simulink model "Geneva_Drive"  (R2017a)
settings: Solver=ode15s  StartTime=0.0  StopTime=30  MaxStep=1e-2  RelTol=1e-4  AbsTol=1e-5  EnableMultiTasking=on
PostLoadFcn:
  | set_param(bdroot,'IgnoredZcDiagnostic','none')
  | warning off sm:compiler:topologyAnalysis:DanglingBlock
StartFcn:
  | tic;
StopFcn:
  | Elapsed_Sim_Time = toc;
  | disp(['Elapsed Sim Time = ' num2str(Elapsed_Sim_Time)]);
undefined symbols (not defined in the file or in its folder): X, Y, Z
libraries: sm_lib x44, Contact_Forces_Lib x20, nesl_utility x5, simulink x1
(part 1 of 2)
CloseFcn:
  | try,close(h1_Geneva_Drive),end
  | clear h1_Geneva_Drive
  | 
  | clear simlog_Geneva_Drive
Description:
  | Geneva Drive
  | 
  | Copyright 2015-2017 The MathWorks, Inc.
settings Model: Creator=smiller  LastModifiedBy=smiller
settings DataIOCC: MaxDataPoints=15000  SaveFormat=StructureWithTime  SaveState=on  SignalLoggingName=logsout_Geneva_Drive
settings OptimizationCC: LifeSpan=inf
settings DebuggingCC: IgnoredZcDiagnostic=none  SolverPrmCheckMsg=warning  AllowSymbolicDim=off  SFUnexpectedBacktrackingDiag=warning  SFNoUnconditionalDefaultTransitionDiag=warning  SFExecutionAtInitializationDiag=none
settings HardwareCC: ProdBitPerPointer=32  ProdBitPerSizeT=32  ProdBitPerPtrDiffT=32  ProdLargestAtomicFloat=None  ProdIntDivRoundTo=Undefined  ProdEndianess=Unspecified  ProdWordSize=32  ProdHWDeviceType=32-bit Generic
settings ModelReferenceCC: PropagateSignalLabelsOutOfModel=off
settings GRTTargetCC: TargetLangStandard=C89/C90 (ANSI)  GeneratePreprocessorConditionals=Disable all
settings ConfigComp: CovMetricSettings=dw  CovHtmlReporting=on  CovSaveCumulativeToWorkspaceVar=on  CovSaveSingleToWorkspaceVar=on  CovExternalEMLEnable=off  CovSFcnEnable=off
settings SimscapeCC: SimscapeLogType=all  SimscapeLogSimulationStatistics=on  SimscapeLogName=simlog_Geneva_Drive  SimscapeLogDataHistory=15000
settings ConfigurationSet: Description=SimMechanics 2G
settings ExplorerConfigSet: InternalSimMechanicsExplorerSettings="<ExplorerConfiguration><canonicalview>default</canonicalview><AnimationSetting><BasePlaybackSpeed>1.0</BasePlaybackSpeed><PlaybackSpeedFactor>4.0</PlaybackSpeedFactor></AnimationSetting><TilePanel><TileInfo><Tiles Columns=\"1\" Count=\"1\" Rows=\"1\"><Column Left=\"2\" Weight=\"1\"/><Column Left=\"677\"/><Row Top=\"2\" Weight=\"1\"/><Row Top=\"558\"/><Tile Height=\"1\" Width=\"1\" X=\"0\" Y=\"0\"/></Tiles></TileInfo><SceneInfo><SceneViewer><BGColor><R>0.93725490570068359</R><G>0.9686274528503418</G><B>0.9686274528503418</B></BGColor><Camera><Position><X>0.26080521668652706</X><Y>0.4639017710068058</Y><Z>0.36701914488687676</Z></Position><Center><X>-0.034093618327655228</X><Y>0.025639318022065816</Y><Z>-0.010275526182887462</Z></Center><Up><X>-0.45579088703273962</X><Y>0.73671340761661774</Y><Z>-0.4995077800553458</Z></Up><Left>-0.33774445205926895</Left><Right>0.33774445205926895</Right><Bottom>-0.208832748234272</Bottom><Top>0.208832748234272</Top></Camera></SceneViewer></SceneInfo></TilePanel></ExplorerConfiguration>"

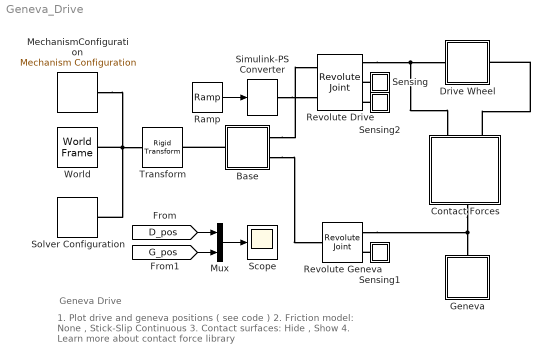
== system Geneva_Drive ==
  note: 1. Plot drive and geneva positions ( see code )
      | 2. Friction model: None , Stick-Slip Continuous
      | 3. Contact surfaces: Hide , Show
      | 4. Learn more about contact force library
  note: Geneva Drive
  Base : Subsystem
  Contact Forces : Subsystem
  Drive Wheel : Subsystem  Tag=CustomStyle
  Geneva : Subsystem  Tag=CustomStyle
  MechanismConfiguration : sm_lib/Utilities/Mechanism Configuration  UniformGravity=Constant  GravityVector=[0 -9.81 0]  GravityUnits=m/s^2  LinearizationDelta=0.001
  Mux : Mux  Inputs=2
  Ramp : simulink/Sources/Ramp  slope=72  start=0  X0=106.26478005487978
  Revolute Drive : sm_lib/Joints/Revolute Joint  SenseConstraintForce=off  SenseConstraintForceX=off  SenseConstraintForceY=off  SenseConstraintForceZ=off  SenseConstraintTorque=off  SenseConstraintTorqueX=off  SenseConstraintTorqueY=off  SenseConstraintTorqueZ=off  SenseTotalForce=off  SenseTotalForceX=off  SenseTotalForceY=off  SenseTotalForceZ=off  SenseTotalTorque=off  SenseTotalTorqueX=off  SenseTotalTorqueY=off  SenseTotalTorqueZ=off  CompositeWrenchDir=FollowerOnBase  CompositeWrenchFrame=BaseFrame  EquilibriumPosition=0  EquilibriumPositionUnits=rad  SpringStiffness=0  SpringStiffnessUnits=m*N/rad  DampingCoefficient=0  DampingCoefficientUnits=m*s*N/rad  TorqueActuationMode=ComputedTorque  MotionActuationMode=InputMotion  SensePosition=on  SenseVelocity=off  SenseAcceleration=off  SenseTorqueForce=on  PositionTargetSpecify=on  PositionTargetPriority=Low  PositionTargetValue=106.26478005487978  PositionTargetValueUnits=deg  VelocityTargetSpecify=off  VelocityTargetPriority=High  VelocityTargetValue=0  VelocityTargetValueUnits=deg/s
  Revolute Geneva : sm_lib/Joints/Revolute Joint  SenseConstraintForce=off  SenseConstraintForceX=off  SenseConstraintForceY=off  SenseConstraintForceZ=off  SenseConstraintTorque=off  SenseConstraintTorqueX=off  SenseConstraintTorqueY=off  SenseConstraintTorqueZ=off  SenseTotalForce=off  SenseTotalForceX=off  SenseTotalForceY=off  SenseTotalForceZ=off  SenseTotalTorque=off  SenseTotalTorqueX=off  SenseTotalTorqueY=off  SenseTotalTorqueZ=off  CompositeWrenchDir=FollowerOnBase  CompositeWrenchFrame=BaseFrame  EquilibriumPosition=90.000000000003197  EquilibriumPositionUnits=deg  SpringStiffness=0  SpringStiffnessUnits=m*N/rad  DampingCoefficient=1  DampingCoefficientUnits=m*s*N/rad  TorqueActuationMode=NoTorque  MotionActuationMode=ComputedMotion  SensePosition=on  SenseVelocity=off  SenseAcceleration=off  SenseTorqueForce=off  PositionTargetSpecify=on  PositionTargetPriority=Low  PositionTargetValue=90.000000000003197  PositionTargetValueUnits=deg  VelocityTargetSpecify=off  VelocityTargetPriority=High  VelocityTargetValue=0  VelocityTargetValueUnits=deg/s
  Scope : Scope
  Sensing : Subsystem  Tag=CustomStyle
  Sensing1 : Subsystem  Tag=CustomStyle
  Sensing2 : Subsystem
  Simulink-PS Converter : nesl_utility/Simulink-PS Converter  PhysicalDomain=network_engine_domain  SubClassName=ps_input  LeftPortType=input  RightPortType=output  PseudoPeriodic=off  Frequencies=[]  NoiseDistribution=none  NoiseParameters=[]  Unit=deg  AffineConversion=off  FilteringAndDerivatives=filter  SimscapeFilterOrder=2  InputFilterTimeConstant=0.01  UdotUserProvided=1
  Solver Configuration : nesl_utility/Solver Configuration  PhysicalDomain=network_engine_domain  SubClassName=solver  LeftPortType=input  RightPortType=generic  Accelerate=off  Tones=[]  Harmonics=[]  SimulateNoise=off  Profile=off  UseLocalSampling=off  EnableSwitchedLinearOptims=on  FrequencyDomain=off  UseCCode=off  RelTol=0.001  AbsTol=1e-06  MinStep=1e-09  ToWorkspace=off  RevertToSquareIcSolve=off  NumHomotopyIterations=100  PhasorMode=off  PhasorModeNumHarmonics=1  OverrideAbsTol=off  DoDC=off  ResidualTolerance=1e-09  UseLocalSolver=off  LocalSolverChoice=NE_BACKWARD_EULER_ADVANCER  LocalSolverSampleTime=0.001  DoFixedCost=off  MaxNonlinIter=3  MaxModeIter=2  LinearAlgebra=Sparse  DelaysMemoryBudget=1024  AutomaticFiltering=on  FilteringTimeConstant=0.001
  "Transform " : sm_lib/Frames and Transforms/Rigid Transform  TranslationMethod=Cartesian  TranslationStandardOffset=0  TranslationLengthUnit=mm  TranslationStandardAxis=+Z  TranslationCartesianOffset=[-30.994181557875464 40 -14.83110487348719]  TranslationROffset=0  TranslationROffsetUnits=m  TranslationZOffset=0  TranslationZOffsetUnits=m  TranslationThetaOffset=0  TranslationThetaOffsetUnits=deg  RotationMethod=ArbitraryAxis  RotationAngleUnits=rad  RotationStandardAxis=+Z  RotationAngle=1.5707963267948966  RotationArbitraryAxis=[-1 0 0]  FollAlignAxisA=+X  BaseAlignAxisA=+Y  FollAlignAxisB=+Y  BaseAlignAxisB=+Z  RotationSequenceAxes=FollowerAxes  RotationSequence=XYX  RotationSequenceAngles=[0 0 0]  RotationSequenceAnglesUnits=deg  RotationMatrix=[1 0 0; 0 1 0; 0 0 1]
  World : sm_lib/Frames and Transforms/World Frame
  wires:
  Ramp/1 -> Simulink-PS Converter/1
  [D_pos] -> Mux/1
  Mux/1 -> Scope/1
  [G_pos] -> Mux/2
  connections:
  World/RConn1 -- MechanismConfiguration/RConn1 -- "Transform "/LConn1 -- Solver Configuration/RConn1
  Revolute Drive/RConn1 -- Drive Wheel/LConn1 -- Contact Forces/RConn1
  Revolute Geneva/RConn1 -- Geneva/LConn1 -- Contact Forces/LConn1
  Sensing2/LConn1 -- Revolute Drive/RConn3
  Sensing1/LConn1 -- Revolute Geneva/RConn2
  Sensing/LConn1 -- Revolute Drive/RConn2
  Contact Forces/RConn2 -- Drive Wheel/RConn1
  Simulink-PS Converter/RConn1 -- Revolute Drive/LConn2
  Base/LConn1 -- "Transform "/RConn1
  Base/RConn1 -- Revolute Drive/LConn1
  Base/RConn2 -- Revolute Geneva/LConn1

== system Geneva_Drive/Base ==
  ReferenceFrame : sm_lib/Frames and Transforms/Reference Frame
  Solid : sm_lib/Body Elements/Solid  InertiaType=Custom  Mass=5.6121441650895836  MassUnits=kg  CenterOfMass=[0.22415415704528135 0 -24.782168314450626]  CenterOfMassUnits=mm  MomentsOfInertia=[57246.923822174664 131168.16755878026 187513.90774897448]  MomentsOfInertiaUnits=kg*mm^2  ProductsOfInertia=[0 -24.879239071091789 0]  ProductsOfInertiaUnits=kg*mm^2  DensityBased=on  Density=1000  DensityUnits=kg/(m^3)  DoExposeReferenceFrame=on  SerializedFrames=<Frames/>  GraphicType=FromGeometry  MarkerShape=Sphere  MarkerSize=10  MarkerSizeUnits=m  GraphicVisPropType=SimpleVisualProperties  GraphicDiffuseColor=[0.82745098039215681 0.82745098039215681 0.81960784313725488]  GraphicSpecularColor=[0.5 0.5 0.5 1.0]  GraphicAmbientColor=[0.15 0.15 0.15 1.0]  GraphicEmissiveColor=[0.0 0.0 0.0 1.0]  GraphicShininess=75  GraphicOpacity=1  GeometryShape=FromFile  RectangleSize=[1 1]  RectangleSizeUnits=m  BrickDimensions=[1 1 1]  BrickDimensionUnits=m  CylinderRadius=1  CylinderRadiusUnits=m  CylinderLength=1  CylinderLengthUnits=m  SphereRadius=1  SphereRadiusUnits=m  EllipsoidRadii=[1 1 1]  EllipsoidRadiiUnits=m  ExtrusionCrossSection=[1 1; -1 1; -1 -1; 1 -1]  ExtrusionCrossSectionUnits=m  ExtrusionLength=1  ExtrusionLengthUnits=m  PolygonNumSides=3  PolygonOuterRadius=1  PolygonOuterRadiusUnits=m  ExtGeomFileType=STL  ExtGeomFileName=Base_Default_sldprt.STL  ExtGeomFileUnits=mm  RevolutionCrossSection=[1 1; 1 -1; 2 -1; 2 1]  RevolutionCrossSectionUnits=m  RevolutionExtent=Full  RevolutionAngle=180  RevolutionAngleUnits=deg
  Transform : sm_lib/Frames and Transforms/Rigid Transform  TranslationMethod=Cartesian  TranslationStandardOffset=0  TranslationLengthUnit=mm  TranslationStandardAxis=+Z  TranslationCartesianOffset=[100 0 0]  TranslationROffset=0  TranslationROffsetUnits=m  TranslationZOffset=0  TranslationZOffsetUnits=m  TranslationThetaOffset=0  TranslationThetaOffsetUnits=deg  RotationMethod=ArbitraryAxis  RotationAngleUnits=rad  RotationStandardAxis=+Z  RotationAngle=0  RotationArbitraryAxis=[0 0 0]  FollAlignAxisA=+X  BaseAlignAxisA=+Y  FollAlignAxisB=+Y  BaseAlignAxisB=+Z  RotationSequenceAxes=FollowerAxes  RotationSequence=XYX  RotationSequenceAngles=[0 0 0]  RotationSequenceAnglesUnits=deg  RotationMatrix=[1 0 0; 0 1 0; 0 0 1]
  Transform2 : sm_lib/Frames and Transforms/Rigid Transform  TranslationMethod=Cartesian  TranslationStandardOffset=0  TranslationLengthUnit=mm  TranslationStandardAxis=+Z  TranslationCartesianOffset=[-99.999999999999986 0 57.42640687119286*0]  TranslationROffset=0  TranslationROffsetUnits=m  TranslationZOffset=0  TranslationZOffsetUnits=m  TranslationThetaOffset=0  TranslationThetaOffsetUnits=deg  RotationMethod=ArbitraryAxis  RotationAngleUnits=rad  RotationStandardAxis=+Z  RotationAngle=3.1415926535897931  RotationArbitraryAxis=[1 0 0]  FollAlignAxisA=+X  BaseAlignAxisA=+Y  FollAlignAxisB=+Y  BaseAlignAxisB=+Z  RotationSequenceAxes=FollowerAxes  RotationSequence=XYX  RotationSequenceAngles=[0 0 0]  RotationSequenceAnglesUnits=deg  RotationMatrix=[1 0 0; 0 1 0; 0 0 1]
  F3 : PMIOPort  Port=1  Side=Left
  F2 : PMIOPort  Port=2  Side=Right
  F : PMIOPort  Port=3  Side=Right
  connections:
  Transform2/RConn1 -- F2/RConn1
  Transform/RConn1 -- F/RConn1
  F3/RConn1 -- Transform2/LConn1 -- Transform/LConn1 -- ReferenceFrame/RConn1 -- Solid/RConn1

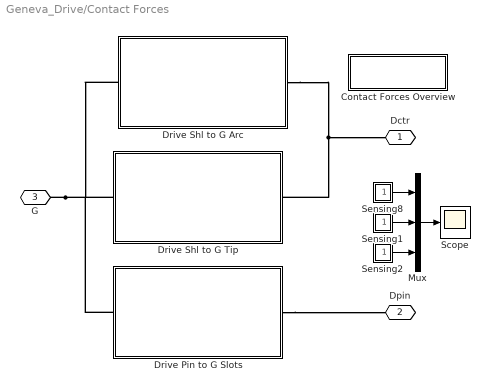
== system Geneva_Drive/Contact Forces ==
  Contact Forces Overview : Subsystem
      settings: OpenFcn=web(which('Geneva_Drive_Contact_Forces.html'));
      mask Display: disp('Contact Forces\nOverview');
  Drive Pin to G Slots : Subsystem  mask(Contact Forces, Drive Pin and Geneva Slot){r_drive_pin=0.015, l_genv_lin=0.1405*2, k_contact=1e5, b_contact=1e4, d_genv_lin=0.0055, vis_len_genevadrive=0.03, vis_dep_genevadrive=0.001}
      mask prompts: r_drive_pin "Radius of Drive Wheel Pin (m)"; l_genv_lin "Slot Length Through Geneva (m)"; k_contact "Contact Stiffness (N/m)"; b_contact "Contact Damping (N/(m/s))"; d_genv_lin "Line Thickness, Geneva Slot (m)"; vis_len_genevadrive "Contact Surface Visualization Height(m)"; vis_dep_genevadrive "Contact Surface Visualization Thickness (m)"
      mask help:
      | This subsystem models the contact forces between the drive wheel pin and the four slots on the Geneva.  All contact forces are identical.  They connect one reference frame on the drive wheel pin and four reference frames on the Geneva.
      |
      | Click the Help button for a diagram of the contact forces and the parameters.
      mask Help: web(which('Geneva_Drive_Contact_DPin_GSlot.html'));
      mask Display:
      | image(imread('Contact_Diagram_Dpin_to_GSlot_IMAGE.jpg'));
      | port_label('LConn',1,'LinB');
      | port_label('RConn',1,'CirF');
  Drive Shl to G Arc : Subsystem  mask(Contact Forces, Drive Shoulder and Geneva Arc){r_shld_cir=0.005, r_genv_xcir=0.115, d_genv_ctr_to_xcir=0.2, k_contact=1e4, b_contact=1e2, d_genv_xcir=0.005, vis_len_genevadrive=0.03, vis_dep_genevadrive=0.001}
      mask prompts: r_shld_cir "Circle Radius, Drive Wheel Shoulder (m)"; r_genv_xcir "Ring Radius, Geneva Arc (m)"; d_genv_ctr_to_xcir "Distance Geneva axis to center exterior circle (m)"; k_contact "Contact Stiffness (N/m)"; b_contact "Contact Damping (N/(m/s))"; d_genv_xcir "Ring Thickness, Geneva Arc (m)"; vis_len_genevadrive "Contact Surface Visualization Height(m)"; vis_dep_genevadrive "Contact Surface Visualization Thickness (m)"
      mask help:
      | This subsystem models the contact forces between the drive wheel shoulder and the exterior arcs on the Geneva.  All contact forces are identical.  They connect two reference frames on the drive wheel and four reference frames on the Geneva.
      |
      | Click the Help button for a diagram of the contact forces and the parameters.
      mask Help: web(which('Geneva_Drive_Contact_Shld_Garc.html'));
      mask Display:
      | image(imread('Contact_Diagram_Shld_to_GArc_IMAGE.jpg'));
      | port_label('Lconn',1,'RinB');
      | port_label('Rconn',1,'CirF');
  Drive Shl to G Tip : Subsystem  mask(Contact Forces, Drive Shoulder and Geneva Tips){r_genv_cir=0.0045, r_shld=0.115, k_contact=1e4, b_contact=1e2, d_shld=0.005, vis_len_genevadrive=0.03, vis_dep_genevadrive=0.001}
      mask prompts: r_genv_cir "Circle Radius, Geneva Tip Contact (m)"; r_shld "Ring Radius, Drive Wheel Shoulder (m)"; k_contact "Contact Stiffness (N/m)"; b_contact "Contact Damping (N/(m/s))"; d_shld "Ring Thickness, Drive Wheel Shoulder (m)"; vis_len_genevadrive "Contact Surface Visualization Height(m)"; vis_dep_genevadrive "Contact Surface Visualization Thickness (m)"
      mask help:
      | This subsystem models the contact forces between the drive wheel shoulder and the tips of the Geneva.  All contact forces are identical.  They connect one reference frame on the drive wheel and eight reference frames on the Geneva.
      |
      | Click the Help button for a diagram of the contact forces and the parameters.
      mask Help: web(which('Geneva_Drive_Contact_Shld_Gtip.html'));
      mask Display:
      | image(imread('Contact_Diagram_Gtip_to_Shld_IMAGE.jpg'));
      | port_label('Lconn',1,'CirF');
      | port_label('Rconn',1,'RinB');
  Mux : Mux  Inputs=3
  Scope : Scope
  Sensing1 : Subsystem
  Sensing2 : Subsystem
  Sensing8 : Subsystem
  Dctr : PMIOPort  Port=1  Side=Right
  Dpin : PMIOPort  Port=2  Side=Right
  G : PMIOPort  Port=3  Side=Left
  wires:
  Mux/1 -> Scope/1
  Sensing2/1(S) -> Mux/3
  Sensing1/1(S) -> Mux/2
  Sensing8/1(S) -> Mux/1
  connections:
  G/RConn1 -- Drive Shl to G Arc/LConn1 -- Drive Pin to G Slots/LConn1 -- Drive Shl to G Tip/LConn1
  Drive Pin to G Slots/RConn1 -- Dpin/RConn1
  Drive Shl to G Arc/RConn1 -- Dctr/RConn1 -- Drive Shl to G Tip/RConn1

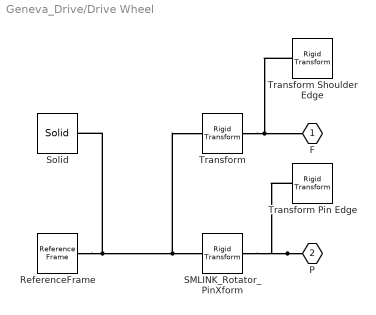
== system Geneva_Drive/Drive Wheel ==
  ReferenceFrame : sm_lib/Frames and Transforms/Reference Frame
  SMLINK_Rotator_PinXform : sm_lib/Frames and Transforms/Rigid Transform  TranslationMethod=Cartesian  TranslationStandardOffset=0  TranslationLengthUnit=mm  TranslationStandardAxis=+Z  TranslationCartesianOffset=[0 99.999999999999943 1.0000000000000009]  TranslationROffset=0  TranslationROffsetUnits=m  TranslationZOffset=0  TranslationZOffsetUnits=m  TranslationThetaOffset=0  TranslationThetaOffsetUnits=deg  RotationMethod=StandardAxis  RotationAngleUnits=deg  RotationStandardAxis=+Z  RotationAngle=10  RotationArbitraryAxis=[0 0 1]  FollAlignAxisA=+X  BaseAlignAxisA=+Y  FollAlignAxisB=+Y  BaseAlignAxisB=+Z  RotationSequenceAxes=FollowerAxes  RotationSequence=XYX  RotationSequenceAngles=[0 0 0]  RotationSequenceAnglesUnits=deg  RotationMatrix=[1 0 0; 0 1 0; 0 0 1]
  Solid : sm_lib/Body Elements/Solid  InertiaType=Custom  Mass=1.1459440199505517  MassUnits=kg  CenterOfMass=[-103.32572655678197 -3.3257265567819814 0.56035000006051983]  CenterOfMassUnits=mm  MomentsOfInertia=[5063.1142307875289 5063.1142307875298 10008.151794093599]  MomentsOfInertiaUnits=kg*mm^2  ProductsOfInertia=[46.956086417341879 46.956086417341901 41.94861289102812]  ProductsOfInertiaUnits=kg*mm^2  DensityBased=on  Density=1000  DensityUnits=kg/(m^3)  DoExposeReferenceFrame=on  SerializedFrames=<Frames/>  GraphicType=FromGeometry  MarkerShape=Sphere  MarkerSize=10  MarkerSizeUnits=m  GraphicVisPropType=SimpleVisualProperties  GraphicDiffuseColor=[0.2 0.4 1.0]  GraphicSpecularColor=[0.5 0.5 0.5 1.0]  GraphicAmbientColor=[0.15 0.15 0.15 1.0]  GraphicEmissiveColor=[0.0 0.0 0.0 1.0]  GraphicShininess=75  GraphicOpacity=1  GeometryShape=FromFile  RectangleSize=[1 1]  RectangleSizeUnits=m  BrickDimensions=[1 1 1]  BrickDimensionUnits=m  CylinderRadius=1  CylinderRadiusUnits=m  CylinderLength=1  CylinderLengthUnits=m  SphereRadius=1  SphereRadiusUnits=m  EllipsoidRadii=[1 1 1]  EllipsoidRadiiUnits=m  ExtrusionCrossSection=[1 1; -1 1; -1 -1; 1 -1]  ExtrusionCrossSectionUnits=m  ExtrusionLength=1  ExtrusionLengthUnits=m  PolygonNumSides=3  PolygonOuterRadius=1  PolygonOuterRadiusUnits=m  ExtGeomFileType=STL  ExtGeomFileName=Drive_Wheel_Default_sldprt.STL  ExtGeomFileUnits=mm  RevolutionCrossSection=[1 1; 1 -1; 2 -1; 2 1]  RevolutionCrossSectionUnits=m  RevolutionExtent=Full  RevolutionAngle=180  RevolutionAngleUnits=deg
  Transform : sm_lib/Frames and Transforms/Rigid Transform  TranslationMethod=Cartesian  TranslationStandardOffset=0  TranslationLengthUnit=mm  TranslationStandardAxis=+Z  TranslationCartesianOffset=[-100.00000000000026 2.1316282072803006e-14 57.426406871192782*0]  TranslationROffset=0  TranslationROffsetUnits=m  TranslationZOffset=0  TranslationZOffsetUnits=m  TranslationThetaOffset=0  TranslationThetaOffsetUnits=deg  RotationMethod=ArbitraryAxis  RotationAngleUnits=rad  RotationStandardAxis=+Z  RotationAngle=3.1415926535897931  RotationArbitraryAxis=[-1 5.9163189700902024e-33 -6.6609835156154749e-17]  FollAlignAxisA=+X  BaseAlignAxisA=+Y  FollAlignAxisB=+Y  BaseAlignAxisB=+Z  RotationSequenceAxes=FollowerAxes  RotationSequence=XYX  RotationSequenceAngles=[0 0 0]  RotationSequenceAnglesUnits=deg  RotationMatrix=[1 0 0; 0 1 0; 0 0 1]
  Transform Pin Edge : sm_lib/Frames and Transforms/Rigid Transform  TranslationMethod=StandardAxis  TranslationStandardOffset=0.015  TranslationLengthUnit=m  TranslationStandardAxis=+X  TranslationCartesianOffset=[0 0 0]  TranslationROffset=0.115  TranslationROffsetUnits=m  TranslationZOffset=0  TranslationZOffsetUnits=m  TranslationThetaOffset=270  TranslationThetaOffsetUnits=deg  RotationMethod=None  RotationAngleUnits=deg  RotationStandardAxis=+Z  RotationAngle=0  RotationArbitraryAxis=[0 0 1]  FollAlignAxisA=+X  BaseAlignAxisA=+Y  FollAlignAxisB=+Y  BaseAlignAxisB=+Z  RotationSequenceAxes=FollowerAxes  RotationSequence=XYX  RotationSequenceAngles=[0 0 0]  RotationSequenceAnglesUnits=deg  RotationMatrix=[1 0 0; 0 1 0; 0 0 1]
  Transform Shoulder Edge : sm_lib/Frames and Transforms/Rigid Transform  TranslationMethod=Cylindrical  TranslationStandardOffset=0.115  TranslationLengthUnit=m  TranslationStandardAxis=+X  TranslationCartesianOffset=[0 0 0]  TranslationROffset=0.115  TranslationROffsetUnits=m  TranslationZOffset=0  TranslationZOffsetUnits=m  TranslationThetaOffset=270  TranslationThetaOffsetUnits=deg  RotationMethod=None  RotationAngleUnits=deg  RotationStandardAxis=+Z  RotationAngle=0  RotationArbitraryAxis=[0 0 1]  FollAlignAxisA=+X  BaseAlignAxisA=+Y  FollAlignAxisB=+Y  BaseAlignAxisB=+Z  RotationSequenceAxes=FollowerAxes  RotationSequence=XYX  RotationSequenceAngles=[0 0 0]  RotationSequenceAnglesUnits=deg  RotationMatrix=[1 0 0; 0 1 0; 0 0 1]
  F : PMIOPort  Port=1  Side=Left
  P : PMIOPort  Port=2  Side=Right
  connections:
  Transform Shoulder Edge/LConn1 -- F/RConn1 -- Transform/RConn1
  P/RConn1 -- Transform Pin Edge/LConn1 -- SMLINK_Rotator_PinXform/RConn1
  ReferenceFrame/RConn1 -- Solid/RConn1 -- Transform/LConn1 -- SMLINK_Rotator_PinXform/LConn1

== system Geneva_Drive/Geneva ==
  ReferenceFrame : sm_lib/Frames and Transforms/Reference Frame
  Solid : sm_lib/Body Elements/Solid  InertiaType=Custom  Mass=0.24105441419713447  MassUnits=kg  CenterOfMass=[100.00000000000023 1.1564451014440063e-12 5.0000000000000009]  CenterOfMassUnits=mm  MomentsOfInertia=[803.62795532691052 803.62795532691234 1603.261580672231]  MomentsOfInertiaUnits=kg*mm^2  ProductsOfInertia=[0 0 0]  ProductsOfInertiaUnits=kg*mm^2  DensityBased=on  Density=1000  DensityUnits=kg/(m^3)  DoExposeReferenceFrame=on  SerializedFrames=<Frames/>  GraphicType=FromGeometry  MarkerShape=Sphere  MarkerSize=10  MarkerSizeUnits=m  GraphicVisPropType=SimpleVisualProperties  GraphicDiffuseColor=[1.0 0.4 0.0]  GraphicSpecularColor=[0.5 0.5 0.5 1.0]  GraphicAmbientColor=[0.15 0.15 0.15 1.0]  GraphicEmissiveColor=[0.0 0.0 0.0 1.0]  GraphicShininess=75  GraphicOpacity=1  GeometryShape=FromFile  RectangleSize=[1 1]  RectangleSizeUnits=m  BrickDimensions=[1 1 1]  BrickDimensionUnits=m  CylinderRadius=1  CylinderRadiusUnits=m  CylinderLength=1  CylinderLengthUnits=m  SphereRadius=1  SphereRadiusUnits=m  EllipsoidRadii=[1 1 1]  EllipsoidRadiiUnits=m  ExtrusionCrossSection=[1 1; -1 1; -1 -1; 1 -1]  ExtrusionCrossSectionUnits=m  ExtrusionLength=1  ExtrusionLengthUnits=m  PolygonNumSides=3  PolygonOuterRadius=1  PolygonOuterRadiusUnits=m  ExtGeomFileType=STL  ExtGeomFileName=Geneva_Default_sldprt.STL  ExtGeomFileUnits=mm  RevolutionCrossSection=[1 1; 1 -1; 2 -1; 2 1]  RevolutionCrossSectionUnits=m  RevolutionExtent=Full  RevolutionAngle=180  RevolutionAngleUnits=deg
  Transform Ref to Ctr : sm_lib/Frames and Transforms/Rigid Transform  TranslationMethod=Cartesian  TranslationStandardOffset=0  TranslationLengthUnit=mm  TranslationStandardAxis=+Z  TranslationCartesianOffset=[99.999999999999261 -2.4158453015843406e-13 -1.4210854715202004e-14]  TranslationROffset=0  TranslationROffsetUnits=m  TranslationZOffset=0  TranslationZOffsetUnits=m  TranslationThetaOffset=0  TranslationThetaOffsetUnits=deg  RotationMethod=ArbitraryAxis  RotationAngleUnits=rad  RotationStandardAxis=+Z  RotationAngle=0  RotationArbitraryAxis=[0 0 0]  FollAlignAxisA=+X  BaseAlignAxisA=+Y  FollAlignAxisB=+Y  BaseAlignAxisB=+Z  RotationSequenceAxes=FollowerAxes  RotationSequence=XYX  RotationSequenceAngles=[0 0 0]  RotationSequenceAnglesUnits=deg  RotationMatrix=[1 0 0; 0 1 0; 0 0 1]
  F : PMIOPort  Port=1  Side=Left
  connections:
  F/RConn1 -- Transform Ref to Ctr/RConn1
  Transform Ref to Ctr/LConn1 -- ReferenceFrame/RConn1 -- Solid/RConn1

== system Geneva_Drive/Sensing ==
  PS-Simulink Converter : nesl_utility/PS-Simulink Converter  PhysicalDomain=network_engine_domain  SubClassName=ps_output  LeftPortType=input  RightPortType=output  PseudoPeriodic=off  Frequencies=[]  Unit=rev  AffineConversion=off
  S : PMIOPort  Port=1  Side=Left
  tag scope: D_pos=global
  wires:
  PS-Simulink Converter/1 -> [D_pos]
  connections:
  PS-Simulink Converter/LConn1 -- S/RConn1

== system Geneva_Drive/Sensing1 ==
  PS-Simulink Converter : nesl_utility/PS-Simulink Converter  PhysicalDomain=network_engine_domain  SubClassName=ps_output  LeftPortType=input  RightPortType=output  PseudoPeriodic=off  Frequencies=[]  Unit=rev  AffineConversion=off
  S : PMIOPort  Port=1  Side=Left
  tag scope: G_pos=global
  wires:
  PS-Simulink Converter/1 -> [G_pos]
  connections:
  PS-Simulink Converter/LConn1 -- S/RConn1

== system Geneva_Drive/Sensing2 ==
  PS-Simulink Converter : nesl_utility/PS-Simulink Converter  PhysicalDomain=network_engine_domain  SubClassName=ps_output  LeftPortType=input  RightPortType=output  PseudoPeriodic=off  Frequencies=[]  Unit=1  AffineConversion=off
  Required Torque : Scope
  S : PMIOPort  Port=1  Side=Left
  wires:
  PS-Simulink Converter/1 -> Required Torque/1
  connections:
  PS-Simulink Converter/LConn1 -- S/RConn1

== system Geneva_Drive/Contact Forces/Contact Forces Overview ==

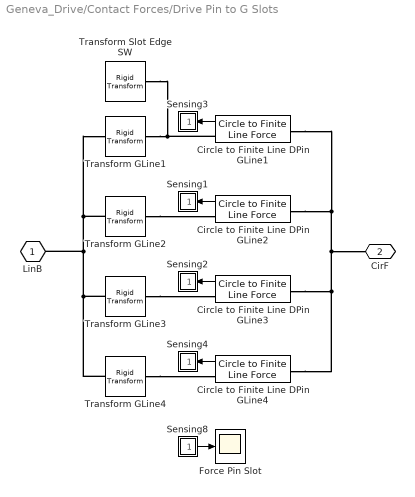
== system Geneva_Drive/Contact Forces/Drive Pin to G Slots ==
  Circle to Finite Line DPin GLine{1..4} (4 alike) : Contact_Forces_Lib/2D/Circle to Finite Line Force  circle_rad=r_drive_pin  line_depth=d_genv_lin  line_length=l_genv_lin  force_law=Linear  k_contact=k_contact  b_contact=b_contact  pen_full_damp_F=1e-4  pen_exponent=1  custom_param_1=1  custom_param_2=1  friction_law=None  mu_kinetic=0.5  mu_static=0.7  v_thr=0.001  vis_on=off  vis_opc_en=0  vis_len_linBz=vis_len_genevadrive  vis_len_linBx=vis_dep_genevadrive  vis_len_cirFz=vis_len_genevadrive  vis_len_cirFx=vis_dep_genevadrive  vis_clr=[0.9 0.2 0.2]  vis_opc=0.7
      settings: SourceProductName=Simscape Multibody Contact Forces Library
  Force Pin Slot : Scope
  Sensing1 : Subsystem
  Sensing2 : Subsystem
  Sensing3 : Subsystem
  Sensing4 : Subsystem
  Sensing8 : Subsystem
  Transform GLine1 : sm_lib/Frames and Transforms/Rigid Transform  TranslationMethod=Cylindrical  TranslationStandardOffset=0  TranslationLengthUnit=m  TranslationStandardAxis=+Z  TranslationCartesianOffset=[0 0 0]  TranslationROffset=-0.02  TranslationROffsetUnits=m  TranslationZOffset=0  TranslationZOffsetUnits=m  TranslationThetaOffset=315  TranslationThetaOffsetUnits=deg  RotationMethod=StandardAxis  RotationAngleUnits=deg  RotationStandardAxis=+Z  RotationAngle=315  RotationArbitraryAxis=[0 0 1]  FollAlignAxisA=+X  BaseAlignAxisA=+Y  FollAlignAxisB=+Y  BaseAlignAxisB=+Z  RotationSequenceAxes=FollowerAxes  RotationSequence=XYX  RotationSequenceAngles=[0 0 0]  RotationSequenceAnglesUnits=deg  RotationMatrix=[1 0 0; 0 1 0; 0 0 1]
  Transform GLine2 : sm_lib/Frames and Transforms/Rigid Transform  TranslationMethod=Cylindrical  TranslationStandardOffset=0  TranslationLengthUnit=m  TranslationStandardAxis=+Z  TranslationCartesianOffset=[0 0 0]  TranslationROffset=-0.02  TranslationROffsetUnits=m  TranslationZOffset=0  TranslationZOffsetUnits=m  TranslationThetaOffset=135  TranslationThetaOffsetUnits=deg  RotationMethod=StandardAxis  RotationAngleUnits=deg  RotationStandardAxis=+Z  RotationAngle=135  RotationArbitraryAxis=[0 0 1]  FollAlignAxisA=+X  BaseAlignAxisA=+Y  FollAlignAxisB=+Y  BaseAlignAxisB=+Z  RotationSequenceAxes=FollowerAxes  RotationSequence=XYX  RotationSequenceAngles=[0 0 0]  RotationSequenceAnglesUnits=deg  RotationMatrix=[1 0 0; 0 1 0; 0 0 1]
  Transform GLine3 : sm_lib/Frames and Transforms/Rigid Transform  TranslationMethod=Cylindrical  TranslationStandardOffset=0  TranslationLengthUnit=m  TranslationStandardAxis=+Z  TranslationCartesianOffset=[0 0 0]  TranslationROffset=-0.02  TranslationROffsetUnits=m  TranslationZOffset=0  TranslationZOffsetUnits=m  TranslationThetaOffset=225  TranslationThetaOffsetUnits=deg  RotationMethod=StandardAxis  RotationAngleUnits=deg  RotationStandardAxis=+Z  RotationAngle=225  RotationArbitraryAxis=[0 0 1]  FollAlignAxisA=+X  BaseAlignAxisA=+Y  FollAlignAxisB=+Y  BaseAlignAxisB=+Z  RotationSequenceAxes=FollowerAxes  RotationSequence=XYX  RotationSequenceAngles=[0 0 0]  RotationSequenceAnglesUnits=deg  RotationMatrix=[1 0 0; 0 1 0; 0 0 1]
  Transform GLine4 : sm_lib/Frames and Transforms/Rigid Transform  TranslationMethod=Cylindrical  TranslationStandardOffset=0  TranslationLengthUnit=m  TranslationStandardAxis=+Z  TranslationCartesianOffset=[0 0 0]  TranslationROffset=-0.02  TranslationROffsetUnits=m  TranslationZOffset=0  TranslationZOffsetUnits=m  TranslationThetaOffset=45  TranslationThetaOffsetUnits=deg  RotationMethod=StandardAxis  RotationAngleUnits=deg  RotationStandardAxis=+Z  RotationAngle=45  RotationArbitraryAxis=[0 0 1]  FollAlignAxisA=+X  BaseAlignAxisA=+Y  FollAlignAxisB=+Y  BaseAlignAxisB=+Z  RotationSequenceAxes=FollowerAxes  RotationSequence=XYX  RotationSequenceAngles=[0 0 0]  RotationSequenceAnglesUnits=deg  RotationMatrix=[1 0 0; 0 1 0; 0 0 1]
  Transform Slot Edge SW : sm_lib/Frames and Transforms/Rigid Transform  TranslationMethod=StandardAxis  TranslationStandardOffset=0.005  TranslationLengthUnit=m  TranslationStandardAxis=+X  TranslationCartesianOffset=[0 0 0]  TranslationROffset=0  TranslationROffsetUnits=m  TranslationZOffset=0  TranslationZOffsetUnits=m  TranslationThetaOffset=0  TranslationThetaOffsetUnits=deg  RotationMethod=None  RotationAngleUnits=deg  RotationStandardAxis=+Z  RotationAngle=45  RotationArbitraryAxis=[0 0 1]  FollAlignAxisA=+X  BaseAlignAxisA=+Y  FollAlignAxisB=+Y  BaseAlignAxisB=+Z  RotationSequenceAxes=FollowerAxes  RotationSequence=XYX  RotationSequenceAngles=[0 0 0]  RotationSequenceAnglesUnits=deg  RotationMatrix=[1 0 0; 0 1 0; 0 0 1]
  LinB : PMIOPort  Port=1  Side=Left
  CirF : PMIOPort  Port=2  Side=Right
  wires:
  Sensing8/1(S) -> Force Pin Slot/1
  Circle to Finite Line DPin GLine4/1 -> Sensing4/1(S)
  Circle to Finite Line DPin GLine3/1 -> Sensing2/1(S)
  Circle to Finite Line DPin GLine2/1 -> Sensing1/1(S)
  Circle to Finite Line DPin GLine1/1 -> Sensing3/1(S)
  connections:
  Transform GLine2/RConn1 -- Circle to Finite Line DPin GLine2/RConn1
  Transform GLine3/RConn1 -- Circle to Finite Line DPin GLine3/RConn1
  Circle to Finite Line DPin GLine4/LConn1 -- CirF/RConn1 -- Circle to Finite Line DPin GLine2/LConn1 -- Circle to Finite Line DPin GLine1/LConn1 -- Circle to Finite Line DPin GLine3/LConn1
  Transform Slot Edge SW/LConn1 -- Transform GLine1/RConn1 -- Circle to Finite Line DPin GLine1/RConn1
  Transform GLine4/RConn1 -- Circle to Finite Line DPin GLine4/RConn1
  Transform GLine3/LConn1 -- LinB/RConn1 -- Transform GLine2/LConn1 -- Transform GLine1/LConn1 -- Transform GLine4/LConn1

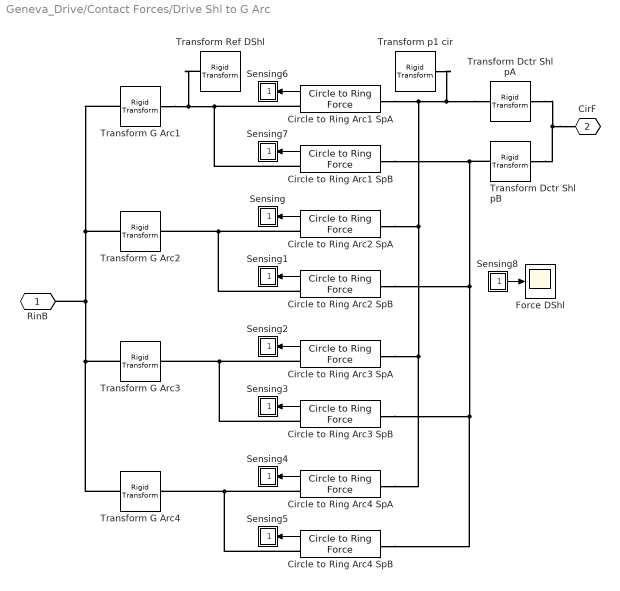
== system Geneva_Drive/Contact Forces/Drive Shl to G Arc ==
  "Circle to Ring Arc1 SpA " : Contact_Forces_Lib/2D/Circle to Ring Force  radius_circle=r_shld_cir  radius_ring=r_genv_xcir+d_genv_xcir/2  d_ring=d_genv_xcir  active_angle=[-45 45]  force_law=Linear  k_contact=k_contact  b_contact=b_contact  pen_full_damp_F=1e-4  pen_exponent=1  custom_param_1=1  custom_param_2=1  friction_law=None  mu_kinetic=0.5  mu_static=0.7  v_thr=0.001  vis_on=off  vis_opc_en=0  vis_len_rinBz=vis_len_genevadrive  vis_len_rinBx=vis_dep_genevadrive  vis_len_cirFz=vis_len_genevadrive  vis_len_cirFx=vis_dep_genevadrive  vis_clr=[0.9 0.2 0.2]  vis_opc=0.7
      settings: SourceProductName=Simscape Multibody Contact Forces Library
  Circle to Ring Arc1 SpB : Contact_Forces_Lib/2D/Circle to Ring Force  radius_circle=r_shld_cir  radius_ring=r_genv_xcir+d_genv_xcir/2  d_ring=d_genv_xcir  active_angle=[-45 45]  force_law=Linear  k_contact=k_contact  b_contact=b_contact  pen_full_damp_F=1e-4  pen_exponent=1  custom_param_1=1  custom_param_2=1  friction_law=None  mu_kinetic=0.5  mu_static=0.7  v_thr=0.001  vis_on=off  vis_opc_en=0  vis_len_rinBz=vis_len_genevadrive  vis_len_rinBx=vis_dep_genevadrive  vis_len_cirFz=vis_len_genevadrive  vis_len_cirFx=vis_dep_genevadrive  vis_clr=[0.9 0.2 0.2]  vis_opc=0.7
      settings: SourceProductName=Simscape Multibody Contact Forces Library
  Circle to Ring Arc2 SpA : Contact_Forces_Lib/2D/Circle to Ring Force  radius_circle=r_shld_cir  radius_ring=r_genv_xcir+d_genv_xcir/2  d_ring=d_genv_xcir  active_angle=[-45 45]  force_law=Linear  k_contact=k_contact  b_contact=b_contact  pen_full_damp_F=1e-4  pen_exponent=1  custom_param_1=1  custom_param_2=1  friction_law=None  mu_kinetic=0.5  mu_static=0.7  v_thr=0.001  vis_on=off  vis_opc_en=0  vis_len_rinBz=vis_len_genevadrive  vis_len_rinBx=vis_dep_genevadrive  vis_len_cirFz=vis_len_genevadrive  vis_len_cirFx=vis_dep_genevadrive  vis_clr=[0.9 0.2 0.2]  vis_opc=0.7
      settings: SourceProductName=Simscape Multibody Contact Forces Library
  Circle to Ring Arc2 SpB : Contact_Forces_Lib/2D/Circle to Ring Force  radius_circle=r_shld_cir  radius_ring=r_genv_xcir+d_genv_xcir/2  d_ring=d_genv_xcir  active_angle=[-45 45]  force_law=Linear  k_contact=k_contact  b_contact=b_contact  pen_full_damp_F=1e-4  pen_exponent=1  custom_param_1=1  custom_param_2=1  friction_law=None  mu_kinetic=0.5  mu_static=0.7  v_thr=0.001  vis_on=off  vis_opc_en=0  vis_len_rinBz=vis_len_genevadrive  vis_len_rinBx=vis_dep_genevadrive  vis_len_cirFz=vis_len_genevadrive  vis_len_cirFx=vis_dep_genevadrive  vis_clr=[0.9 0.2 0.2]  vis_opc=0.7
      settings: SourceProductName=Simscape Multibody Contact Forces Library
  Circle to Ring Arc3 SpA : Contact_Forces_Lib/2D/Circle to Ring Force  radius_circle=r_shld_cir  radius_ring=r_genv_xcir+d_genv_xcir/2  d_ring=d_genv_xcir  active_angle=[-45 45]  force_law=Linear  k_contact=k_contact  b_contact=b_contact  pen_full_damp_F=1e-4  pen_exponent=1  custom_param_1=1  custom_param_2=1  friction_law=None  mu_kinetic=0.5  mu_static=0.7  v_thr=0.001  vis_on=off  vis_opc_en=0  vis_len_rinBz=vis_len_genevadrive  vis_len_rinBx=vis_dep_genevadrive  vis_len_cirFz=vis_len_genevadrive  vis_len_cirFx=vis_dep_genevadrive  vis_clr=[0.9 0.2 0.2]  vis_opc=0.7
      settings: SourceProductName=Simscape Multibody Contact Forces Library
  Circle to Ring Arc3 SpB : Contact_Forces_Lib/2D/Circle to Ring Force  radius_circle=r_shld_cir  radius_ring=r_genv_xcir+d_genv_xcir/2  d_ring=d_genv_xcir  active_angle=[-45 45]  force_law=Linear  k_contact=k_contact  b_contact=b_contact  pen_full_damp_F=1e-4  pen_exponent=1  custom_param_1=1  custom_param_2=1  friction_law=None  mu_kinetic=0.5  mu_static=0.7  v_thr=0.001  vis_on=off  vis_opc_en=0  vis_len_rinBz=vis_len_genevadrive  vis_len_rinBx=vis_dep_genevadrive  vis_len_cirFz=vis_len_genevadrive  vis_len_cirFx=vis_dep_genevadrive  vis_clr=[0.9 0.2 0.2]  vis_opc=0.7
      settings: SourceProductName=Simscape Multibody Contact Forces Library
  Circle to Ring Arc4 SpA : Contact_Forces_Lib/2D/Circle to Ring Force  radius_circle=r_shld_cir  radius_ring=r_genv_xcir+d_genv_xcir/2  d_ring=d_genv_xcir  active_angle=[-45 45]  force_law=Linear  k_contact=k_contact  b_contact=b_contact  pen_full_damp_F=1e-4  pen_exponent=1  custom_param_1=1  custom_param_2=1  friction_law=None  mu_kinetic=0.5  mu_static=0.7  v_thr=0.001  vis_on=off  vis_opc_en=0  vis_len_rinBz=vis_len_genevadrive  vis_len_rinBx=vis_dep_genevadrive  vis_len_cirFz=vis_len_genevadrive  vis_len_cirFx=vis_dep_genevadrive  vis_clr=[0.9 0.2 0.2]  vis_opc=0.7
      settings: SourceProductName=Simscape Multibody Contact Forces Library
  Circle to Ring Arc4 SpB : Contact_Forces_Lib/2D/Circle to Ring Force  radius_circle=r_shld_cir  radius_ring=r_genv_xcir+d_genv_xcir/2  d_ring=d_genv_xcir  active_angle=[-45 45]  force_law=Linear  k_contact=k_contact  b_contact=b_contact  pen_full_damp_F=1e-4  pen_exponent=1  custom_param_1=1  custom_param_2=1  friction_law=None  mu_kinetic=0.5  mu_static=0.7  v_thr=0.001  vis_on=off  vis_opc_en=0  vis_len_rinBz=vis_len_genevadrive  vis_len_rinBx=vis_dep_genevadrive  vis_len_cirFz=vis_len_genevadrive  vis_len_cirFx=vis_dep_genevadrive  vis_clr=[0.9 0.2 0.2]  vis_opc=0.7
      settings: SourceProductName=Simscape Multibody Contact Forces Library
  Force DShl : Scope
  Sensing : Subsystem
  Sensing1 : Subsystem
  Sensing2 : Subsystem
  Sensing3 : Subsystem
  Sensing4 : Subsystem
  Sensing5 : Subsystem
  Sensing6 : Subsystem
  Sensing7 : Subsystem
  Sensing8 : Subsystem
  Transform Dctr Shl pA : sm_lib/Frames and Transforms/Rigid Transform  TranslationMethod=StandardAxis  TranslationStandardOffset=r_genv_xcir-r_shld_cir  TranslationLengthUnit=m  TranslationStandardAxis=+X  TranslationCartesianOffset=[0 0 0]  TranslationROffset=0  TranslationROffsetUnits=m  TranslationZOffset=0  TranslationZOffsetUnits=m  TranslationThetaOffset=0  TranslationThetaOffsetUnits=deg  RotationMethod=None  RotationAngleUnits=deg  RotationStandardAxis=+X  RotationAngle=180  RotationArbitraryAxis=[0 0 1]  FollAlignAxisA=+X  BaseAlignAxisA=+Y  FollAlignAxisB=+Y  BaseAlignAxisB=+Z  RotationSequenceAxes=FollowerAxes  RotationSequence=XYX  RotationSequenceAngles=[0 0 0]  RotationSequenceAnglesUnits=deg  RotationMatrix=[1 0 0; 0 1 0; 0 0 1]
  Transform Dctr Shl pB : sm_lib/Frames and Transforms/Rigid Transform  TranslationMethod=StandardAxis  TranslationStandardOffset=r_genv_xcir-r_shld_cir  TranslationLengthUnit=m  TranslationStandardAxis=-Y  TranslationCartesianOffset=[0 0 0]  TranslationROffset=0  TranslationROffsetUnits=m  TranslationZOffset=0  TranslationZOffsetUnits=m  TranslationThetaOffset=0  TranslationThetaOffsetUnits=deg  RotationMethod=None  RotationAngleUnits=deg  RotationStandardAxis=+Z  RotationAngle=180  RotationArbitraryAxis=[0 0 1]  FollAlignAxisA=+X  BaseAlignAxisA=+Y  FollAlignAxisB=+Y  BaseAlignAxisB=+Z  RotationSequenceAxes=FollowerAxes  RotationSequence=XYX  RotationSequenceAngles=[0 0 0]  RotationSequenceAnglesUnits=deg  RotationMatrix=[1 0 0; 0 1 0; 0 0 1]
  Transform G Arc1 : sm_lib/Frames and Transforms/Rigid Transform  TranslationMethod=StandardAxis  TranslationStandardOffset=d_genv_ctr_to_xcir  TranslationLengthUnit=m  TranslationStandardAxis=+Y  TranslationCartesianOffset=[0 0 0]  TranslationROffset=0  TranslationROffsetUnits=m  TranslationZOffset=0  TranslationZOffsetUnits=m  TranslationThetaOffset=0  TranslationThetaOffsetUnits=deg  RotationMethod=StandardAxis  RotationAngleUnits=deg  RotationStandardAxis=+Z  RotationAngle=-90  RotationArbitraryAxis=[0 0 1]  FollAlignAxisA=+X  BaseAlignAxisA=+Y  FollAlignAxisB=+Y  BaseAlignAxisB=+Z  RotationSequenceAxes=FollowerAxes  RotationSequence=XYX  RotationSequenceAngles=[0 0 0]  RotationSequenceAnglesUnits=deg  RotationMatrix=[1 0 0; 0 1 0; 0 0 1]
  Transform G Arc2 : sm_lib/Frames and Transforms/Rigid Transform  TranslationMethod=StandardAxis  TranslationStandardOffset=d_genv_ctr_to_xcir  TranslationLengthUnit=m  TranslationStandardAxis=+X  TranslationCartesianOffset=[0 0 0]  TranslationROffset=0  TranslationROffsetUnits=m  TranslationZOffset=0  TranslationZOffsetUnits=m  TranslationThetaOffset=0  TranslationThetaOffsetUnits=deg  RotationMethod=StandardAxis  RotationAngleUnits=deg  RotationStandardAxis=+Z  RotationAngle=180  RotationArbitraryAxis=[0 0 1]  FollAlignAxisA=+X  BaseAlignAxisA=+Y  FollAlignAxisB=+Y  BaseAlignAxisB=+Z  RotationSequenceAxes=FollowerAxes  RotationSequence=XYX  RotationSequenceAngles=[0 0 0]  RotationSequenceAnglesUnits=deg  RotationMatrix=[1 0 0; 0 1 0; 0 0 1]
  Transform G Arc3 : sm_lib/Frames and Transforms/Rigid Transform  TranslationMethod=StandardAxis  TranslationStandardOffset=d_genv_ctr_to_xcir  TranslationLengthUnit=m  TranslationStandardAxis=-Y  TranslationCartesianOffset=[0 0 0]  TranslationROffset=0  TranslationROffsetUnits=m  TranslationZOffset=0  TranslationZOffsetUnits=m  TranslationThetaOffset=0  TranslationThetaOffsetUnits=deg  RotationMethod=StandardAxis  RotationAngleUnits=deg  RotationStandardAxis=+Z  RotationAngle=90  RotationArbitraryAxis=[0 0 1]  FollAlignAxisA=+X  BaseAlignAxisA=+Y  FollAlignAxisB=+Y  BaseAlignAxisB=+Z  RotationSequenceAxes=FollowerAxes  RotationSequence=XYX  RotationSequenceAngles=[0 0 0]  RotationSequenceAnglesUnits=deg  RotationMatrix=[1 0 0; 0 1 0; 0 0 1]
  Transform G Arc4 : sm_lib/Frames and Transforms/Rigid Transform  TranslationMethod=StandardAxis  TranslationStandardOffset=d_genv_ctr_to_xcir  TranslationLengthUnit=m  TranslationStandardAxis=-X  TranslationCartesianOffset=[0 0 0]  TranslationROffset=0  TranslationROffsetUnits=m  TranslationZOffset=0  TranslationZOffsetUnits=m  TranslationThetaOffset=0  TranslationThetaOffsetUnits=deg  RotationMethod=StandardAxis  RotationAngleUnits=deg  RotationStandardAxis=+Z  RotationAngle=0  RotationArbitraryAxis=[0 0 1]  FollAlignAxisA=+X  BaseAlignAxisA=+Y  FollAlignAxisB=+Y  BaseAlignAxisB=+Z  RotationSequenceAxes=FollowerAxes  RotationSequence=XYX  RotationSequenceAngles=[0 0 0]  RotationSequenceAnglesUnits=deg  RotationMatrix=[1 0 0; 0 1 0; 0 0 1]
  Transform Ref DShl : sm_lib/Frames and Transforms/Rigid Transform  TranslationMethod=StandardAxis  TranslationStandardOffset=r_genv_xcir  TranslationLengthUnit=m  TranslationStandardAxis=+X  TranslationCartesianOffset=[0 0 0]  TranslationROffset=0  TranslationROffsetUnits=m  TranslationZOffset=0  TranslationZOffsetUnits=m  TranslationThetaOffset=0  TranslationThetaOffsetUnits=deg  RotationMethod=None  RotationAngleUnits=deg  RotationStandardAxis=+Z  RotationAngle=0  RotationArbitraryAxis=[0 0 1]  FollAlignAxisA=+X  BaseAlignAxisA=+Y  FollAlignAxisB=+Y  BaseAlignAxisB=+Z  RotationSequenceAxes=FollowerAxes  RotationSequence=XYX  RotationSequenceAngles=[0 0 0]  RotationSequenceAnglesUnits=deg  RotationMatrix=[1 0 0; 0 1 0; 0 0 1]
  Transform p1 cir : sm_lib/Frames and Transforms/Rigid Transform  TranslationMethod=StandardAxis  TranslationStandardOffset=r_shld_cir  TranslationLengthUnit=m  TranslationStandardAxis=+X  TranslationCartesianOffset=[0 0 0]  TranslationROffset=0  TranslationROffsetUnits=m  TranslationZOffset=0  TranslationZOffsetUnits=m  TranslationThetaOffset=0  TranslationThetaOffsetUnits=deg  RotationMethod=None  RotationAngleUnits=deg  RotationStandardAxis=+Z  RotationAngle=0  RotationArbitraryAxis=[0 0 1]  FollAlignAxisA=+X  BaseAlignAxisA=+Y  FollAlignAxisB=+Y  BaseAlignAxisB=+Z  RotationSequenceAxes=FollowerAxes  RotationSequence=XYX  RotationSequenceAngles=[0 0 0]  RotationSequenceAnglesUnits=deg  RotationMatrix=[1 0 0; 0 1 0; 0 0 1]
  RinB : PMIOPort  Port=1  Side=Left
  CirF : PMIOPort  Port=2  Side=Right
  wires:
  Circle to Ring Arc1 SpB/1 -> Sensing7/1(S)
  "Circle to Ring Arc1 SpA "/1 -> Sensing6/1(S)
  Circle to Ring Arc4 SpB/1 -> Sensing5/1(S)
  Circle to Ring Arc4 SpA/1 -> Sensing4/1(S)
  Circle to Ring Arc3 SpB/1 -> Sensing3/1(S)
  Circle to Ring Arc3 SpA/1 -> Sensing2/1(S)
  Circle to Ring Arc2 SpB/1 -> Sensing1/1(S)
  Circle to Ring Arc2 SpA/1 -> Sensing/1(S)
  Sensing8/1(S) -> Force DShl/1
  connections:
  Circle to Ring Arc3 SpA/RConn1 -- Circle to Ring Arc3 SpB/RConn1 -- Transform G Arc3/RConn1
  Transform Dctr Shl pB/RConn1 -- Circle to Ring Arc3 SpB/LConn1 -- Circle to Ring Arc4 SpB/LConn1 -- Circle to Ring Arc2 SpB/LConn1 -- Circle to Ring Arc1 SpB/LConn1
  Circle to Ring Arc4 SpA/RConn1 -- Circle to Ring Arc4 SpB/RConn1 -- Transform G Arc4/RConn1
  Circle to Ring Arc2 SpA/RConn1 -- Circle to Ring Arc2 SpB/RConn1 -- Transform G Arc2/RConn1
  Transform Dctr Shl pA/RConn1 -- Circle to Ring Arc3 SpA/LConn1 -- Circle to Ring Arc4 SpA/LConn1 -- Circle to Ring Arc2 SpA/LConn1 -- "Circle to Ring Arc1 SpA "/LConn1 -- Transform p1 cir/LConn1
  Transform G Arc1/RConn1 -- "Circle to Ring Arc1 SpA "/RConn1 -- Circle to Ring Arc1 SpB/RConn1 -- Transform Ref DShl/LConn1
  RinB/RConn1 -- Transform G Arc3/LConn1 -- Transform G Arc4/LConn1 -- Transform G Arc2/LConn1 -- Transform G Arc1/LConn1
  CirF/RConn1 -- Transform Dctr Shl pA/LConn1 -- Transform Dctr Shl pB/LConn1
